simulink model "sim_nmpc_2020a"  (R2020a)
settings: Solver=VariableStepAuto  StartTime=0.0  StopTime=120  FixedStep=Ts  RelTol=1e-3
values from neighbouring files (symbols this model uses):
  D = zeros(6,6)    [main.m]
  dist_type = 2    [main.m]
  pv = 1    [main.m]
  Vw = 10    [main.m]
libraries: dspadpt3 x1, mpclib x1, simulink x1, aerolibwind2 x1
settings Model: Creator=Kakavand  LastModifiedBy=Kakavand

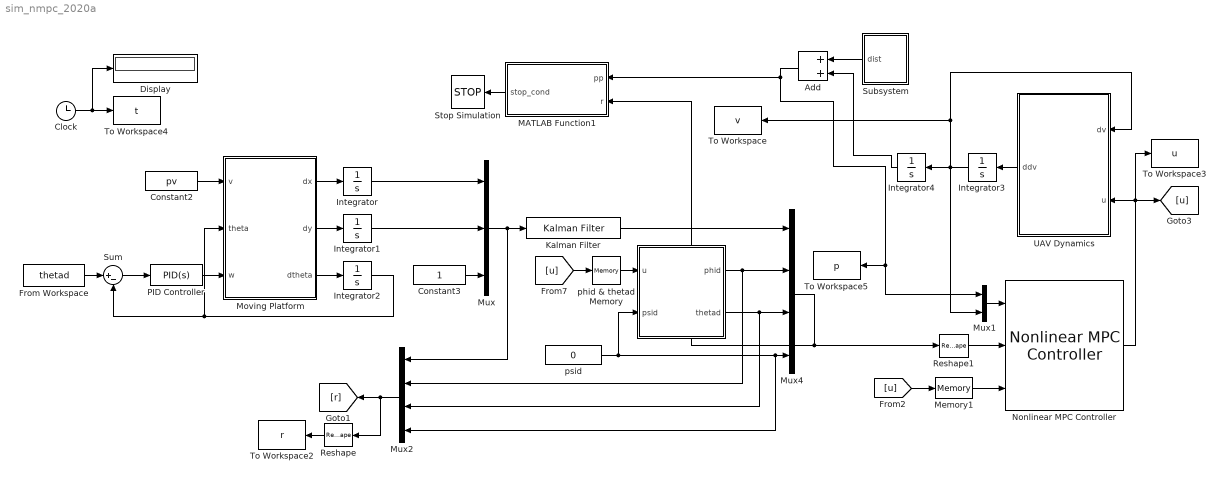
== system sim_nmpc_2020a ==
  Add : Sum
  Clock : Clock
  Constant2 : Constant  Value=pv
  Constant3 : Constant
  Display : Display
  From Workspace : FromWorkspace  VariableName=thetad
  Integrator : Integrator
  Integrator1 : Integrator
  Integrator2 : Integrator
  Integrator3 : Integrator  InitialCondition=[1;-1;1;0;0;0]
  Integrator4 : Integrator  InitialCondition=[3;-3;3;0;0;0]
  Kalman Filter : dspadpt3/Kalman Filter  num_targets=1  sourceEnable=Always  isReset=on  X=zeros([3, 1])  P=10*eye(3)  A=eye(3)  sourceMeasure=Specify via Dialog  H=eye(3)  Q=10*eye(3)  R=eye(3)  isOutputEstMeasure=on  isOutputEstState=off  isOutputEstError=off  isOutputPrdMeasure=off  isOutputPrdState=off  isOutputPrdError=off
      settings: SourceProductBaseCode=DS
  MATLAB Function1 : MATLAB Function  TreatAsAtomicUnit=on
  Memory : Memory  InitialCondition=zeros(6,1)
  Memory1 : Memory  InitialCondition=zeros(6,1)
  Moving Platform : MATLAB Function  TreatAsAtomicUnit=on
  Mux : Mux  Inputs=3
  Mux1 : Mux  Inputs=2
  Mux2 : Mux
  Mux4 : Mux
  Nonlinear MPC Controller : mpclib/Nonlinear MPC Controller  SCDEnableBlockLinearizationSpecification=on  nlmpcobj=nlobj  UseObjectTs=on  UseMEX=off  md_enabled=off  mvtarget_enabled=off  param_enabled=off  cost_enabled=off  mvseq_enabled=off  stateseq_enabled=off  ovseq_enabled=off  slack_enabled=off  status_enabled=off  ov_min=off  ov_max=off  mv_min=off  mv_max=off  mvrate_min=off  mvrate_max=off  state_min=off  state_max=off  ov_weight=off  mv_weight=off  mvrate_weight=off  ecr_weight=off  nlp_initialize=off
  PID Controller : simulink/Continuous/PID Controller  Controller=PID  Form=Parallel  TimeDomain=Continuous-time  UseExternalTs=off  SampleTime=-1  IntegratorMethod=Forward Euler  FilterMethod=Forward Euler  ControllerParametersSource=internal  P=3.9069777102301  I=2.8412915656864  D=-0.21656116417141  UseFilter=on  N=6.54094090429555  TunerSelectOption=Transfer Function Based (PID Tuner App)  InitialConditionSource=internal  InitialConditionForIntegrator=0  InitialConditionForFilter=0  DifferentiatorICPrevScaledInput=0  ExternalReset=none  TrackingMode=off  Kt=1  LimitOutput=off  UpperSaturationLimit=inf  LowerSaturationLimit=-inf  LinearizeAsGain=on  AntiWindupMode=none  Kb=1  POutMin=[]  POutMax=[]  IOutMin=[]  IOutMax=[]  DOutMin=[]  DOutMax=[]  NOutMin=[]  NOutMax=[]  SumOutMin=[]  SumOutMax=[]  SaturationOutMin=[]  SaturationOutMax=[]  PParamMin=[]  PParamMax=[]  IParamMin=[]  IParamMax=[]  DParamMin=[]  DParamMax=[]  NParamMin=[]  NParamMax=[]  KbParamMin=[]  KbParamMax=[]  KtParamMin=[]  KtParamMax=[]  KbOutMin=[]  KbOutMax=[]  KtOutMin=[]  KtOutMax=[]  IntegratorOutMin=[]  IntegratorOutMax=[]  FilterOutMin=[]  FilterOutMax=[]  SumI1OutMin=[]  SumI1OutMax=[]  SumI2OutMin=[]  SumI2OutMax=[]  SumI3OutMin=[]  SumI3OutMax=[]  SumI4OutMin=[]  SumI4OutMax=[]  SumDOutMin=[]  SumDOutMax=[]  DifferentiatorOutMin=[]  DifferentiatorOutMax=[]  FilterDiffOutCoefMin=[]  FilterDiffOutCoefMax=[]  ReciprocalOutMin=[]  ReciprocalOutMax=[]  SumDenOutMin=[]  SumDenOutMax=[]  SumNumOutMin=[]  SumNumOutMax=[]  DivideOutMin=[]  DivideOutMax=[]  UdiffTsProdOutMin=[]  UdiffTsProdOutMax=[]  NTsProdOutMin=[]  NTsProdOutMax=[]  UintegralTsProdOutMin=[]  UintegralTsProdOutMax=[]  UngainTsProdOutMin=[]  UngainTsProdOutMax=[]  IntegratorContinuousStateAttributes=''  IntegratorStateMustResolveToSignalObject=off  IntegratorRTWStateStorageClass=Auto  FilterContinuousStateAttributes=''  FilterStateMustResolveToSignalObject=off  FilterRTWStateStorageClass=Auto  ParallelPVariant=InternalParameters  IdealPVariant=Disabled  IVariant=InternalParameters  DVariant=InternalParameters  IntegratorVariant=Continuous  SatVariant=Disabled  AWVariant=Passthrough  PCopyVariant=Disabled  TRVariant=Disabled  FdbkBlocksVariant=Forward  IdealPFdbkVariant=Disabled  SatFdbkVariant=Disabled  DerivativeFilterVariant=ContFilter  NVariant=InternalParameters  NCopyVariant=Disabled  FilterICVariant=InternalICsFilter  IntegratorICVariant=InternalICs  ExternalResetVariant=Disabled  TRSumVariant=Passthrough  SumFdbkVariant=Disabled  SumVariant=Sum_PID  TsampFilterVariant=InternalTs  TsampNgainVariant=Passthrough  TsampIntegralVariant=Passthrough
  Reshape : Reshape  OutputDimensionality=Row vector (2-D)
  Reshape1 : Reshape  OutputDimensionality=Row vector (2-D)
  Stop Simulation : Stop
  Subsystem : Subsystem
  Sum : Sum  Inputs=|+-
  To Workspace : ToWorkspace  VariableName=v  SampleTime=-1
      settings: Save2DSignal=2-D array (concatenate along first dimension)
  To Workspace2 : ToWorkspace  VariableName=r  SampleTime=-1
      settings: Save2DSignal=2-D array (concatenate along first dimension)
  To Workspace3 : ToWorkspace  VariableName=u  SampleTime=-1
      settings: Save2DSignal=2-D array (concatenate along first dimension)
  To Workspace4 : ToWorkspace  VariableName=t  SampleTime=-1
      settings: Save2DSignal=2-D array (concatenate along first dimension)
  To Workspace5 : ToWorkspace  VariableName=p  SampleTime=-1
      settings: Save2DSignal=2-D array (concatenate along first dimension)
  UAV Dynamics : MATLAB Function  TreatAsAtomicUnit=on
  phid & thetad : MATLAB Function  TreatAsAtomicUnit=on
  psid : Constant  Value=0
  wires:
  Moving Platform/1(dx) -> Integrator/1
  Moving Platform/2(dy) -> Integrator1/1
  Moving Platform/3(dtheta) -> Integrator2/1
  PID Controller/1 -> Moving Platform/3(w)
  Integrator2/1 -> Sum/2, Moving Platform/2(theta)
  Sum/1 -> PID Controller/1
  Constant2/1 -> Moving Platform/1(v)
  From Workspace/1 -> Sum/1
  Integrator/1 -> Mux/1
  Integrator1/1 -> Mux/2
  Mux/1 -> Mux2/1, Kalman Filter/1
  Constant3/1 -> Mux/3
  UAV Dynamics/1(ddv) -> Integrator3/1
  Nonlinear MPC Controller/1 -> To Workspace3/1, UAV Dynamics/2(u), [u]
  Mux4/1 -> Reshape1/1, MATLAB Function1/2(r)
  Kalman Filter/1 -> Mux4/1
  psid/1 -> phid & thetad/2(psid), Mux2/4, Mux4/4
  phid & thetad/2(thetad) -> Mux2/3, Mux4/3
  phid & thetad/1(phid) -> Mux2/2, Mux4/2
  [u] -> Memory/1
  Clock/1 -> Display/1, To Workspace4/1
  Memory/1 -> phid & thetad/1(u)
  Reshape/1 -> To Workspace2/1
  Memory1/1 -> Nonlinear MPC Controller/3
  [u] -> Memory1/1
  Reshape1/1 -> Nonlinear MPC Controller/2
  Mux1/1 -> Nonlinear MPC Controller/1
  Mux2/1 -> Reshape/1, [r]
  Integrator4/1 -> Add/2
  MATLAB Function1/1(stop_cond) -> Stop Simulation/1
  Subsystem/1(dist) -> Add/1
  Integrator3/1 -> Integrator4/1, Mux1/2, UAV Dynamics/1(dv), To Workspace/1
  Add/1 -> MATLAB Function1/1(pp), Mux1/1, To Workspace5/1

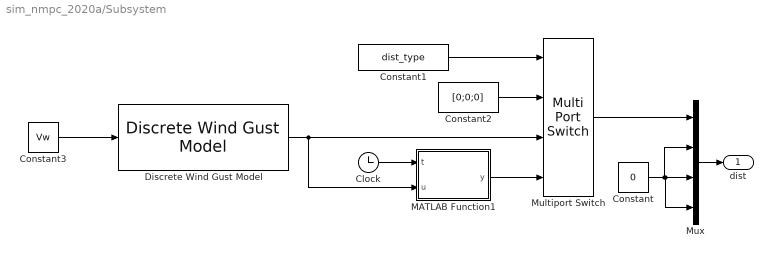
== system sim_nmpc_2020a/Subsystem ==
  Clock : Clock
  Constant : Constant  Value=0
  Constant1 : Constant  Value=dist_type
  Constant2 : Constant  Value=[0;0;0]
  Constant3 : Constant  Value=Vw
  Discrete Wind Gust Model : aerolibwind2/Discrete Wind Gust Model  units=Metric (MKS)  Gx=on  Gy=on  Gz=on  t_0=0  d_m=[120 120 80]  v_m=[3.5 3.5 3.0]
  MATLAB Function1 : MATLAB Function  TreatAsAtomicUnit=on
  Multiport Switch : MultiPortSwitch
  Mux : Mux
  dist : Outport
  wires:
  Constant1/1 -> Multiport Switch/1
  Discrete Wind Gust Model/1 -> MATLAB Function1/2(u), Multiport Switch/3
  Constant2/1 -> Multiport Switch/2
  Constant3/1 -> Discrete Wind Gust Model/1
  MATLAB Function1/1(y) -> Multiport Switch/4
  Clock/1 -> MATLAB Function1/1(t)
  Multiport Switch/1 -> Mux/1
  Constant/1 -> Mux/2, Mux/4, Mux/3
  Mux/1 -> dist/1

== matlab function sim_nmpc_2020a/UAV Dynamics ==
  data: dv input; u input; ddv output
function ddv = fcn(dv,u)
%%  name of states
dx = dv(1);
dy = dv(2);
dz = dv(3);
dphi = dv(4);
dtheta = dv(5);
dpsi = dv(6);

%%  constants
K1 = 1e-3;
K2 = 1e-3;
K3 = 1e-3;
K4 = 1e-3;
K5 = 1e-3;
K6 = 1e-3;
m = 2.85;
Ix = 0.0552;
Iy = 0.0552;
Iz = 0.1104;

%%  dynamics
%   f & g
f_x = -K1/m*dx;
g_x = 1;
%   f & g
f_y = -K2/m*dy;
g_y = 1;
%   f & g
f_z = -K3/m*dz;
g_z = 1;
%   f & g
f_phi = -K4/Ix*dphi + (Iy - Iz)/Ix*dtheta*dpsi;
g_phi = 1/Ix;
%   f & g
f_theta = -K5/Iy*dtheta + (Iz - Ix)/Iy*dphi*dpsi;
g_theta = 1/Iy;
%   f & g
f_psi = -K6/Iz*dpsi + (Ix - Iy)/Iz*dphi*dtheta;
g_psi = 1/Iz;

%%  state eqution
ddv = [f_x+g_x*u(1);f_y+g_y*u(2);f_z+g_z*u(3);...
    f_phi+g_phi*u(4);f_theta+g_theta*u(5);f_psi+g_psi*u(6)];
end

== matlab function sim_nmpc_2020a/Moving Platform ==
  data: v input; theta input; dx output; dy output; dtheta output; w input
function [dx,dy,dtheta] = fcn(v,theta,w)
%   wheel speeds
%  daynamic equations
dx = v/10*cos(theta);
dy = v/10*sin(theta);
dtheta = w;
end

== matlab function sim_nmpc_2020a/MATLAB Function1 ==
  data: pp input; stop_cond output; r input
function stop_cond = fcn(pp,r)
stop_cond = abs(pp(1)-r(1))<=0.2&abs(pp(2)-r(2))<=0.2&abs(pp(3)-r(3))<=0.0005;
end

== matlab function sim_nmpc_2020a/Subsystem/MATLAB Function1 ==
  data: t input; u input; y output
function y = fcn(t,u)
y = u;
if (t > 1)
    y = [0;0;0];
end
end

== matlab function sim_nmpc_2020a/phid & thetad ==
  data: u input; phid output; psid input; thetad output
%%  ALLAH

function [phid,thetad] = fcn(u,psid)
m = 2.85;
g = 9.81;
u_x = u(1); u_y = u(2); u_z = u(3);
u_1 = m*sqrt(u_x^2 + u_y^2 + (u_z+g)^2);
phid = asin(m/u_1*(u_x*sin(psid) - u_y*cos(psid)));
thetad = atan(1/(u_z + g)*(u_x*cos(psid) + u_y*sin(psid)));
end
